simulink subsystem "ideal_regenerator"  (R2022b)
settings: Solver=VariableStepAuto  StartTime=0.0  StopTime=10.0  RelTol=1e-3
undefined symbols (not defined in the file or in its folder): regenerator
libraries: fl_lib x4
settings Model: Creator=wilde  LastModifiedBy=wilde

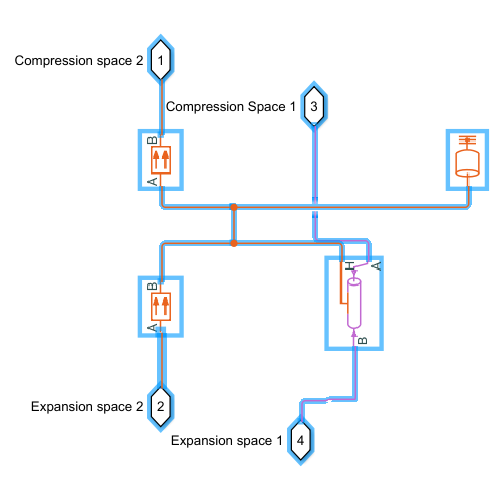
[thumbnail: Simulink's stored preview of the top-level diagram]
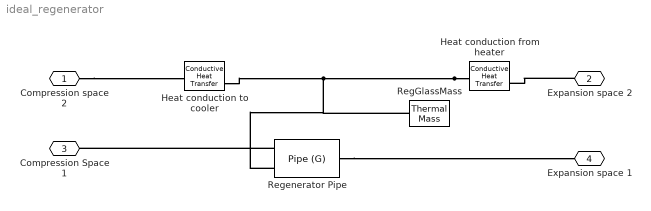
== system ideal_regenerator ==
  Heat conduction from heater : fl_lib/Thermal/Thermal Elements/Conductive Heat Transfer  thermal_type=foundation.enum.ConstantVariableTabulated.Variable  wall_geometry=foundation.enum.ConductionWallGeometry.Planar  area=regenerator.geom.area m^2  thickness=regenerator.Heater.thickness m  d_in=0.05 m  d_out=0.1 m  L=1 m  th_cond_min=10 W/(K*m)  th_cond=regenerator.Heater.k W/(m*K)  th_cond_TLU=[413, 401, 392, 383, 371, 357, 342] W/(K*m)  temp_TLU=[200, 273, 400, 600, 800, 1000, 1200] K  T_specify=off  T_priority=None  T=0 K  T_nominal_specify=off  T_nominal_unit=K  T_nominal_value=1  Q_specify=off  Q_priority=None  Q=0 W  Q_nominal_specify=off  Q_nominal_unit=W  Q_nominal_value=1
      settings: InternalSimscapePortConfiguration="{\"Bottom\":[],\"Left\":[{\"id\":\"A\",\"label\":\"A\",\"type\":\"foundation.thermal.thermal\"},{\"id\":\"var_th_cond\",\"label\":\"K\",\"type\":\"input\"}],\"Right\":[{\"id\":\"B\",\"label\":\"B\",\"type\":\"foundation.thermal.thermal\"}],\"Top\":[]}"
  Heat conduction to cooler : fl_lib/Thermal/Thermal Elements/Conductive Heat Transfer  thermal_type=foundation.enum.ConstantVariableTabulated.Variable  wall_geometry=foundation.enum.ConductionWallGeometry.Planar  area=regenerator.Cooler.area m^2  thickness=regenerator.Cooler.thickness m  d_in=0.05 m  d_out=0.1 m  L=1 m  th_cond_min=10 W/(K*m)  th_cond=regenerator.Cooler.k W/(m*K)  th_cond_TLU=[413, 401, 392, 383, 371, 357, 342] W/(K*m)  temp_TLU=[200, 273, 400, 600, 800, 1000, 1200] K  T_specify=off  T_priority=None  T=0 K  T_nominal_specify=off  T_nominal_unit=K  T_nominal_value=1  Q_specify=off  Q_priority=None  Q=0 W  Q_nominal_specify=off  Q_nominal_unit=W  Q_nominal_value=1
      settings: InternalSimscapePortConfiguration="{\"Bottom\":[],\"Left\":[{\"id\":\"A\",\"label\":\"A\",\"type\":\"foundation.thermal.thermal\"},{\"id\":\"var_th_cond\",\"label\":\"K\",\"type\":\"input\"}],\"Right\":[{\"id\":\"B\",\"label\":\"B\",\"type\":\"foundation.thermal.thermal\"}],\"Top\":[]}"
  RegGlassMass : fl_lib/Thermal/Thermal Elements/Thermal Mass  mass=regenerator.m kg  sp_heat=flame.glass.cp J/kg/K  num_ports=foundation.enum.numPorts2.one  T_specify=on  T_priority=High  T=regenerator.Tinit K  T_nominal_specify=off  T_nominal_unit=K  T_nominal_value=1  Q_specify=off  Q_priority=None  Q=0 W  Q_nominal_specify=off  Q_nominal_unit=W  Q_nominal_value=1
  Regenerator Pipe : fl_lib/Gas/Elements/Pipe (G)  length=regenerator.geom.length m  area=regenerator.geom.area m^2  Dh=regenerator.geom.hydraulic_diam m  length_add=regenerator.therm_fric.length_add m  roughness=regenerator.therm_fric.roughness m  Re_lam=regenerator.therm_fric.Re_lam  Re_tur=regenerator.therm_fric.Re_tur  shape_factor=regenerator.therm_fric.shape_factor  Nu_lam=regenerator.therm_fric.Nu_lam  p_I_specify=on  p_I_priority=High  p_I=state_init.p0 MPa  p_I_nominal_specify=off  p_I_nominal_unit=MPa  p_I_nominal_value=1  T_I_specify=on  T_I_priority=High  T_I=state_init.T0 K  T_I_nominal_specify=off  T_I_nominal_unit=K  T_I_nominal_value=1  rho_pipe_specify=off  rho_pipe_priority=None  rho_pipe=1.2 kg/m^3  rho_pipe_nominal_specify=off  rho_pipe_nominal_unit=kg/m^3  rho_pipe_nominal_value=1
  Compression space 2 : PMIOPort  Side=Left
  Expansion space 2 : PMIOPort  Port=2  Side=Right
  Compression Space 1 : PMIOPort  Port=3  Side=Left
  Expansion space 1 : PMIOPort  Port=4  Side=Right
  connections:
  Heat conduction from heater/RConn1 -- Regenerator Pipe/LConn2 -- RegGlassMass/LConn1 -- Heat conduction to cooler/LConn1
  Regenerator Pipe/LConn1 -- Compression Space 1/RConn1
  Regenerator Pipe/RConn1 -- Expansion space 1/RConn1
  Compression space 2/RConn1 -- Heat conduction to cooler/RConn1
  Expansion space 2/RConn1 -- Heat conduction from heater/LConn1
